simulink model "mini"  (R2023b)
settings: Solver=VariableStepAuto  StartTime=0.0  StopTime=10.0  RelTol=1e-3
libraries: arduinolib x9, arduinosensorlib x1
settings Model: Creator=yeoseojeong  LastModifiedBy=yeoseojeong

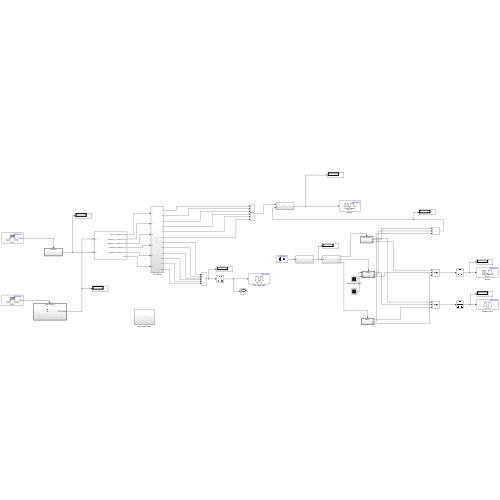
[thumbnail: Simulink's stored preview of the top-level diagram]
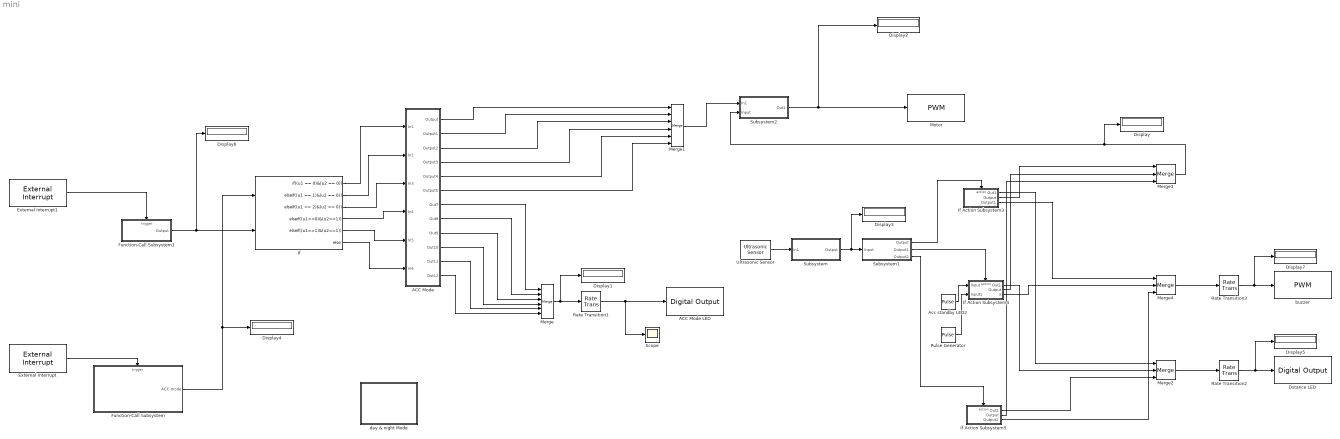
== system mini ==
  ACC Mode : Subsystem
  ACC Mode LED : arduinolib/Digital Output  pinNumber=12  Direction=output  blockPlatform=arduino
  Acc standby LED2 : DiscretePulseGenerator  PulseType=Time based  Period=0.4  PulseWidth=50
  Display{,1..7} (8 alike) : Display
  Dstance LED : arduinolib/Digital Output  pinNumber=13  Direction=output  blockPlatform=arduino
  External Interrupt : arduinolib/External Interrupt  Pin=2  PullUp=off  Mode=RISING  InterruptSimulationInput=off
  External Interrupt1 : arduinolib/External Interrupt  Pin=3  PullUp=off  Mode=RISING  InterruptSimulationInput=off
  Function-Call Subsystem : Subsystem  TreatAsAtomicUnit=on
  Function-Call Subsystem1 : Subsystem  TreatAsAtomicUnit=on
  If : If  NumInputs=2  IfExpression=(u1 == 0)&(u2 == 0)  ElseIfExpressions=(u1 == 1)&(u2 == 0),(u1 == 2)&(u2 == 0),(u1==0)&(u2==1),(u1==1)&(u2==1)
  If Action Subsystem3 : Subsystem  TreatAsAtomicUnit=on
  If Action Subsystem4 : Subsystem  TreatAsAtomicUnit=on
  If Action Subsystem5 : Subsystem  TreatAsAtomicUnit=on
  Merge : Merge  Inputs=6
  Merge1 : Merge  Inputs=6
  Merge2 : Merge  Inputs=3
  Merge3 : Merge  Inputs=3
  Merge4 : Merge  Inputs=3
  Motor : arduinolib/PWM  pinNumber=11  frequencyType=Default  desiredFrequency=490.2  achievableFrequency=490.2
  Pulse Generator : DiscretePulseGenerator  PulseType=Time based  Amplitude=200  PulseWidth=50
  Rate Transition1 : RateTransition  Deterministic=off
  Rate Transition2 : RateTransition  Deterministic=off
  Rate Transition3 : RateTransition  Deterministic=off
  Scope : Scope
  Subsystem : Subsystem
  Subsystem1 : Subsystem
  Subsystem2 : Subsystem
  Ultrasonic Sensor : arduinosensorlib/Ultrasonic Sensor  NumSignalPins=2  TrigPin=50  EchoPin=51  SignalPin=3  SampleTime_=1  blockPlatform=ARDUINO
  buzzer : arduinolib/PWM  pinNumber=5  frequencyType=Default  desiredFrequency=490.2  achievableFrequency=490.1961
  day & night Mode : Subsystem
  wires:
  ACC Mode/6(Output5) -> Merge1/6
  If Action Subsystem5/3(Output1) -> Merge4/3
  ACC Mode/7(Out7) -> Merge/1
  Merge4/1 -> Rate Transition3/1
  Rate Transition3/1 -> buzzer/1, Display7/1
  ACC Mode/8(Out8) -> Merge/2
  ACC Mode/10(Out10) -> Merge/4
  ACC Mode/1(Output) -> Merge1/1
  ACC Mode/12(Out12) -> Merge/6
  Merge2/1 -> Rate Transition2/1
  ACC Mode/9(Out9) -> Merge/3
  ACC Mode/5(Output4) -> Merge1/5
  If/3 -> ACC Mode/3(In3)
  Rate Transition1/1 -> ACC Mode LED/1, Scope/1
  ACC Mode/4(Output3) -> Merge1/4
  If/6 -> ACC Mode/6(In6)
  If/5 -> ACC Mode/5(In5)
  ACC Mode/2(Output1) -> Merge1/2
  If/4 -> ACC Mode/4(In4)
  Merge1/1 -> Subsystem2/1(In1)
  If Action Subsystem4/2(Output) -> Merge3/2
  External Interrupt/1 -> Function-Call Subsystem/Trigger
  If/2 -> ACC Mode/2(In2)
  If Action Subsystem4/3(Output1) -> Merge4/2
  If Action Subsystem3/3(Output1) -> Merge4/1
  Merge/1 -> Display1/1, Rate Transition1/1
  Function-Call Subsystem1/1(Output) -> Display6/1, If/2
  If Action Subsystem5/1(Out1) -> Merge2/3
  ACC Mode/3(Output2) -> Merge1/3
  Subsystem1/3(Output2) -> If Action Subsystem5/Action
  ACC Mode/11(Out11) -> Merge/5
  External Interrupt1/1 -> Function-Call Subsystem1/Trigger
  Pulse Generator/1 -> If Action Subsystem4/2(Input1)
  Acc standby LED2/1 -> If Action Subsystem4/1(Input)
  Merge3/1 -> Subsystem2/2(Input), Display/1
  Rate Transition2/1 -> Display5/1, Dstance LED/1
  If Action Subsystem3/2(Output) -> Merge3/1
  Subsystem1/2(Output1) -> If Action Subsystem4/Action
  Subsystem2/1(Out1) -> Display2/1, Motor/1
  If Action Subsystem3/1(Out1) -> Merge2/1
  Subsystem/1(Output) -> Subsystem1/1(Input), Display3/1
  If Action Subsystem4/1(Out1) -> Merge2/2
  Subsystem1/1(Output) -> If Action Subsystem3/Action
  If/1 -> ACC Mode/1(In1)
  Ultrasonic Sensor/1 -> Subsystem/1(In1)
  Function-Call Subsystem/1(ACC mode) -> Display4/1, If/1
  If Action Subsystem5/2(Output) -> Merge3/3

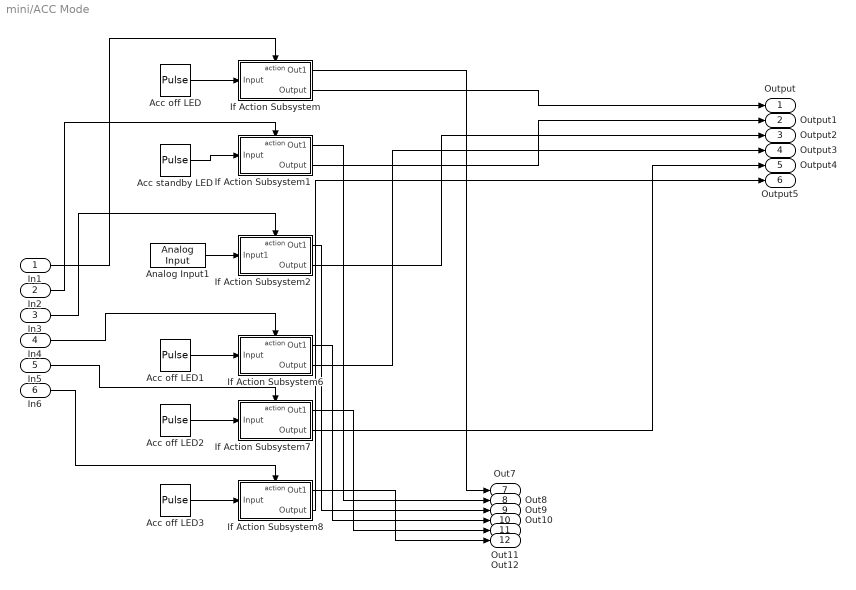
== system mini/ACC Mode ==
  In1 : Inport
  In2 : Inport  Port=2
  In3 : Inport  Port=3
  In4 : Inport  Port=4
  In5 : Inport  Port=5
  In6 : Inport  Port=6
  Acc off LED{,1..3} (4 alike) : DiscretePulseGenerator  PulseType=Time based  PulseWidth=50
  Acc standby LED : DiscretePulseGenerator  PulseType=Time based  Period=0.4  PulseWidth=50
  Analog Input1 : arduinolib/Analog Input  pinNumber=8  ReadResultsOnly=off  ConversionTriggerSource=Software  ExternalTriggerType=uint32( 0 )  OutputDataType=uint16  EnableConversionCompleteNotify=off  EnableOuputStatus=off  SampleTime=-1  blockPlatform=arduino
  If Action Subsystem : Subsystem  TreatAsAtomicUnit=on
  If Action Subsystem1 : Subsystem  TreatAsAtomicUnit=on
  If Action Subsystem2 : Subsystem  TreatAsAtomicUnit=on
  If Action Subsystem6 : Subsystem  TreatAsAtomicUnit=on
  If Action Subsystem7 : Subsystem  TreatAsAtomicUnit=on
  If Action Subsystem8 : Subsystem  TreatAsAtomicUnit=on
  Output : Outport
  Output1 : Outport  Port=2
  Output2 : Outport  Port=3
  Output3 : Outport  Port=4
  Output4 : Outport  Port=5
  Output5 : Outport  Port=6
  Out7 : Outport  Port=7
  Out8 : Outport  Port=8
  Out9 : Outport  Port=9
  Out10 : Outport  Port=10
  Out11 : Outport  Port=11
  Out12 : Outport  Port=12
  wires:
  In2/1 -> If Action Subsystem1/Action
  Acc off LED3/1 -> If Action Subsystem8/1(Input)
  Acc off LED/1 -> If Action Subsystem/1(Input)
  Acc standby LED/1 -> If Action Subsystem1/1(Input)
  If Action Subsystem1/2(Output) -> Output1/1
  If Action Subsystem8/1(Out1) -> Out12/1
  If Action Subsystem2/2(Output) -> Output2/1
  Acc off LED1/1 -> If Action Subsystem6/1(Input)
  Acc off LED2/1 -> If Action Subsystem7/1(Input)
  If Action Subsystem8/2(Output) -> Output5/1
  In3/1 -> If Action Subsystem2/Action
  Analog Input1/1 -> If Action Subsystem2/1(Input1)
  In1/1 -> If Action Subsystem/Action
  If Action Subsystem/1(Out1) -> Out7/1
  If Action Subsystem1/1(Out1) -> Out8/1
  In4/1 -> If Action Subsystem6/Action
  If Action Subsystem6/2(Output) -> Output3/1
  In6/1 -> If Action Subsystem8/Action
  If Action Subsystem/2(Output) -> Output/1
  If Action Subsystem6/1(Out1) -> Out10/1
  If Action Subsystem7/2(Output) -> Output4/1
  If Action Subsystem7/1(Out1) -> Out11/1
  In5/1 -> If Action Subsystem7/Action
  If Action Subsystem2/1(Out1) -> Out9/1

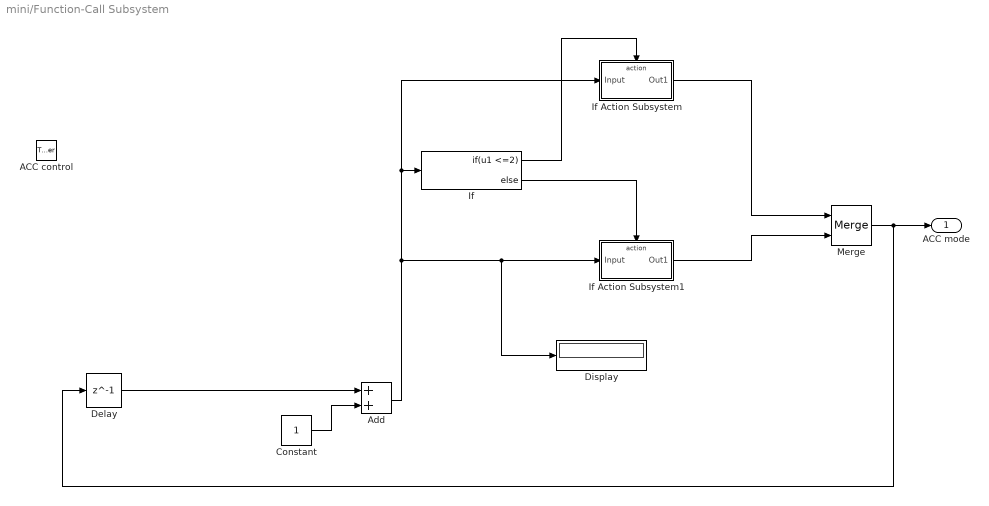
== system mini/Function-Call Subsystem ==
  ACC control : TriggerPort  TriggerType=function-call  VariantControl=(inherit)
  Add : Sum
  Constant : Constant
  Delay : Delay  DelayLength=1
  Display : Display
  If : If  IfExpression=u1 <=2
  If Action Subsystem : Subsystem  TreatAsAtomicUnit=on
  If Action Subsystem1 : Subsystem  TreatAsAtomicUnit=on
  Merge : Merge
  ACC mode : Outport
  wires:
  Delay/1 -> Add/1
  Constant/1 -> Add/2
  If/1 -> If Action Subsystem/Action
  If/2 -> If Action Subsystem1/Action
  If Action Subsystem/1(Out1) -> Merge/1
  If Action Subsystem1/1(Out1) -> Merge/2
  Add/1 -> If Action Subsystem/1(Input), If/1, Display/1, If Action Subsystem1/1(Input)
  Merge/1 -> Delay/1, ACC mode/1

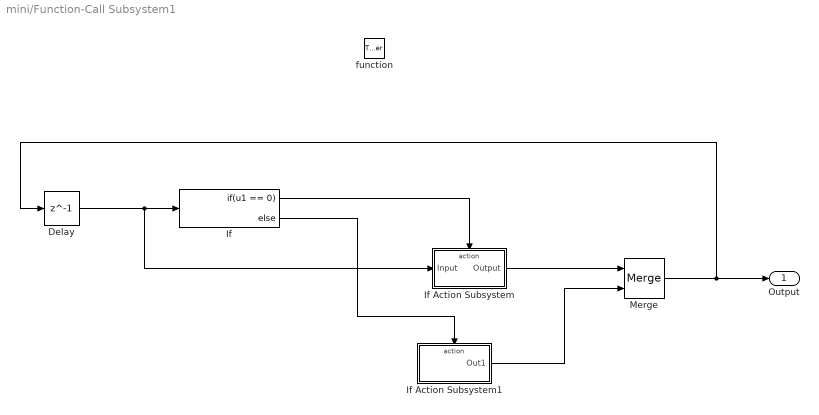
== system mini/Function-Call Subsystem1 ==
  function : TriggerPort  TriggerType=function-call  VariantControl=(inherit)
  Delay : Delay  DelayLength=1
  If : If  IfExpression=u1 == 0
  If Action Subsystem : Subsystem  TreatAsAtomicUnit=on
  If Action Subsystem1 : Subsystem  TreatAsAtomicUnit=on
  Merge : Merge
  Output : Outport
  wires:
  Delay/1 -> If Action Subsystem/1(Input), If/1
  If/1 -> If Action Subsystem/Action
  If Action Subsystem/1(Output) -> Merge/1
  If/2 -> If Action Subsystem1/Action
  If Action Subsystem1/1(Out1) -> Merge/2
  Merge/1 -> Delay/1, Output/1

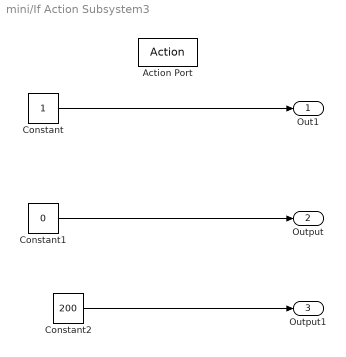
== system mini/If Action Subsystem3 ==
  Action Port : ActionPort  ActionPortLabel=if(u1 <= 200)
  Constant : Constant
  Constant1 : Constant  Value=0
  Constant2 : Constant  Value=200
  Out1 : Outport
  Output : Outport  Port=2
  Output1 : Outport  Port=3
  wires:
  Constant/1 -> Out1/1
  Constant1/1 -> Output/1
  Constant2/1 -> Output1/1

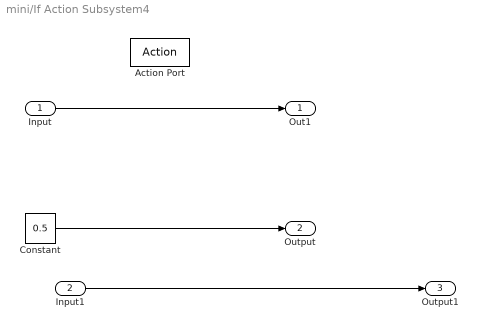
== system mini/If Action Subsystem4 ==
  Input : Inport
  Input1 : Inport  Port=2
  Action Port : ActionPort  ActionPortLabel=elseif(..)
  Constant : Constant  Value=0.5
  Out1 : Outport
  Output : Outport  Port=2
  Output1 : Outport  Port=3
  wires:
  Input/1 -> Out1/1
  Constant/1 -> Output/1
  Input1/1 -> Output1/1

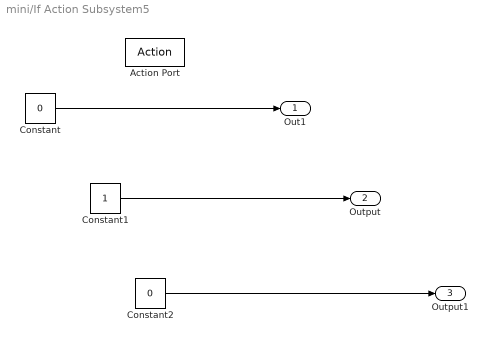
== system mini/If Action Subsystem5 ==
  Action Port : ActionPort  ActionPortLabel=else
  Constant : Constant  Value=0
  Constant1 : Constant
  Constant2 : Constant  Value=0
  Out1 : Outport
  Output : Outport  Port=2
  Output1 : Outport  Port=3
  wires:
  Constant/1 -> Out1/1
  Constant1/1 -> Output/1
  Constant2/1 -> Output1/1

== system mini/Subsystem ==
  In1 : Inport
  Constant : Constant  Value=2
  Constant1 : Constant  Value=3400
  Divide : Product  Inputs=**
  Divide1 : Product  Inputs=*/
  Output : Outport
  wires:
  Constant1/1 -> Divide/2
  Divide/1 -> Divide1/1
  Constant/1 -> Divide1/2
  Divide1/1 -> Output/1
  In1/1 -> Divide/1

== system mini/Subsystem1 ==
  Input : Inport
  If : If  IfExpression=u1 <= 200  ElseIfExpressions=(u1>=250)&(u1<=800)
  Output : Outport
  Output1 : Outport  Port=2
  Output2 : Outport  Port=3
  wires:
  Input/1 -> If/1
  If/1 -> Output/1
  If/2 -> Output1/1
  If/3 -> Output2/1

== system mini/Subsystem2 ==
  In1 : Inport
  Input : Inport  Port=2
  Divide : Product  Inputs=**
  Out1 : Outport
  wires:
  In1/1 -> Divide/1
  Input/1 -> Divide/2
  Divide/1 -> Out1/1

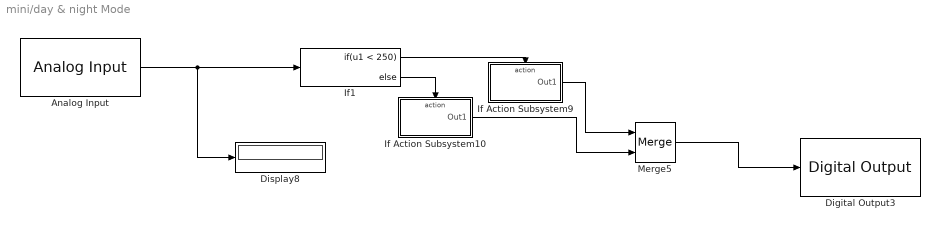
== system mini/day & night Mode ==
  Analog Input : arduinolib/Analog Input  pinNumber=10  ReadResultsOnly=off  ConversionTriggerSource=Software  ExternalTriggerType=uint32( 0 )  OutputDataType=uint16  EnableConversionCompleteNotify=off  EnableOuputStatus=off  SampleTime=-1  blockPlatform=arduino
  Digital Output3 : arduinolib/Digital Output  pinNumber=30  Direction=output  blockPlatform=arduino
  Display8 : Display
  If Action Subsystem10 : Subsystem  TreatAsAtomicUnit=on
  If Action Subsystem9 : Subsystem  TreatAsAtomicUnit=on
  If1 : If  IfExpression=u1 < 250
  Merge5 : Merge
  wires:
  If Action Subsystem10/1(Out1) -> Merge5/2
  If1/2 -> If Action Subsystem10/Action
  Analog Input/1 -> Display8/1, If1/1
  If Action Subsystem9/1(Out1) -> Merge5/1
  If1/1 -> If Action Subsystem9/Action
  Merge5/1 -> Digital Output3/1

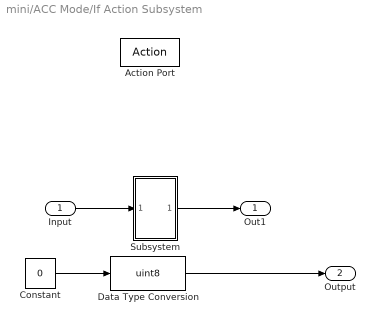
== system mini/ACC Mode/If Action Subsystem ==
  Input : Inport
  Action Port : ActionPort  ActionPortLabel=if((u1 == 0)&(u2 == 0))
  Constant : Constant  Value=0
  Data Type Conversion : DataTypeConversion  OutDataTypeStr=uint8  SaturateOnIntegerOverflow=off  RndMeth=Floor
  Subsystem : Subsystem
  Out1 : Outport
  Output : Outport  Port=2
  wires:
  Constant/1 -> Data Type Conversion/1
  Data Type Conversion/1 -> Output/1
  Input/1 -> Subsystem/1(Input)
  Subsystem/1(Out1) -> Out1/1

== system mini/ACC Mode/If Action Subsystem1 ==
  Input : Inport
  Action Port : ActionPort  ActionPortLabel=elseif((u1 == 1)&(u2 == 0))
  Constant : Constant  Value=120
  Data Type Conversion : DataTypeConversion  OutDataTypeStr=uint8  SaturateOnIntegerOverflow=off  RndMeth=Floor
  Out1 : Outport
  Output : Outport  Port=2
  wires:
  Input/1 -> Out1/1
  Data Type Conversion/1 -> Output/1
  Constant/1 -> Data Type Conversion/1

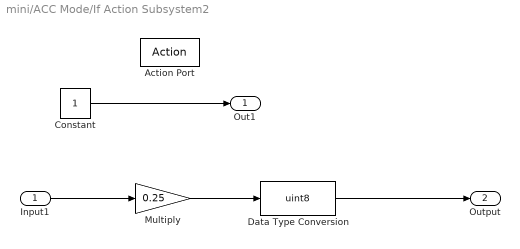
== system mini/ACC Mode/If Action Subsystem2 ==
  Input1 : Inport
  Action Port : ActionPort  ActionPortLabel=elseif((u1 == 2)&(u2 == 0))
  Constant : Constant
  Data Type Conversion : DataTypeConversion  OutDataTypeStr=uint8  SaturateOnIntegerOverflow=off  RndMeth=Floor
  Multiply : Gain  Gain=0.25
  Out1 : Outport
  Output : Outport  Port=2
  wires:
  Constant/1 -> Out1/1
  Input1/1 -> Multiply/1
  Multiply/1 -> Data Type Conversion/1
  Data Type Conversion/1 -> Output/1

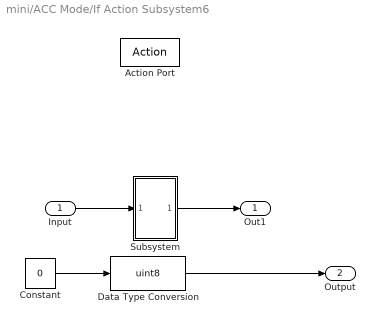
== system mini/ACC Mode/If Action Subsystem6 ==
  Input : Inport
  Action Port : ActionPort  ActionPortLabel=elseif((u1==0)&(u2==1))
  Constant : Constant  Value=0
  Data Type Conversion : DataTypeConversion  OutDataTypeStr=uint8  SaturateOnIntegerOverflow=off  RndMeth=Floor
  Subsystem : Subsystem
  Out1 : Outport
  Output : Outport  Port=2
  wires:
  Constant/1 -> Data Type Conversion/1
  Data Type Conversion/1 -> Output/1
  Input/1 -> Subsystem/1(Input)
  Subsystem/1(Out1) -> Out1/1

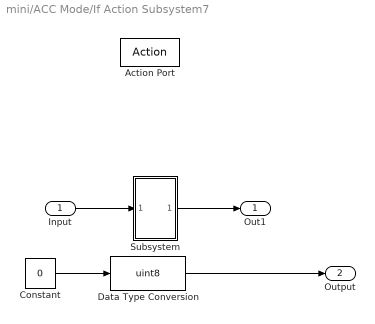
== system mini/ACC Mode/If Action Subsystem7 ==
  Input : Inport
  Action Port : ActionPort  ActionPortLabel=elseif((u1==1)&(u2==1))
  Constant : Constant  Value=0
  Data Type Conversion : DataTypeConversion  OutDataTypeStr=uint8  SaturateOnIntegerOverflow=off  RndMeth=Floor
  Subsystem : Subsystem
  Out1 : Outport
  Output : Outport  Port=2
  wires:
  Constant/1 -> Data Type Conversion/1
  Data Type Conversion/1 -> Output/1
  Input/1 -> Subsystem/1(Input)
  Subsystem/1(Out1) -> Out1/1

== system mini/ACC Mode/If Action Subsystem8 ==
  Input : Inport
  Action Port : ActionPort  ActionPortLabel=else
  Constant : Constant  Value=0
  Data Type Conversion : DataTypeConversion  OutDataTypeStr=uint8  SaturateOnIntegerOverflow=off  RndMeth=Floor
  Subsystem : Subsystem
  Out1 : Outport
  Output : Outport  Port=2
  wires:
  Constant/1 -> Data Type Conversion/1
  Data Type Conversion/1 -> Output/1
  Input/1 -> Subsystem/1(Input)
  Subsystem/1(Out1) -> Out1/1

== system mini/Function-Call Subsystem/If Action Subsystem ==
  Input : Inport
  Action Port : ActionPort  ActionPortLabel=if(u1 <=2)
  Out1 : Outport
  wires:
  Input/1 -> Out1/1

== system mini/Function-Call Subsystem/If Action Subsystem1 ==
  Input : Inport
  Action Port : ActionPort  ActionPortLabel=else
  Constant : Constant  Value=0
  Divide : Product  Inputs=**
  Out1 : Outport
  wires:
  Divide/1 -> Out1/1
  Constant/1 -> Divide/1
  Input/1 -> Divide/2

== system mini/Function-Call Subsystem1/If Action Subsystem ==
  Input : Inport
  Action Port : ActionPort  ActionPortLabel=if(u1 == 0)
  Add : Sum
  Constant : Constant
  Output : Outport
  wires:
  Add/1 -> Output/1
  Input/1 -> Add/1
  Constant/1 -> Add/2

== system mini/Function-Call Subsystem1/If Action Subsystem1 ==
  Action Port : ActionPort  ActionPortLabel=else
  Constant : Constant  Value=0
  Out1 : Outport
  wires:
  Constant/1 -> Out1/1

== system mini/day & night Mode/If Action Subsystem10 ==
  Action Port : ActionPort  ActionPortLabel=else
  Constant : Constant  Value=0
  Out1 : Outport
  wires:
  Constant/1 -> Out1/1

== system mini/day & night Mode/If Action Subsystem9 ==
  Action Port : ActionPort  ActionPortLabel=if(u1 < 250)
  Constant : Constant
  Out1 : Outport
  wires:
  Constant/1 -> Out1/1

== system mini/ACC Mode/If Action Subsystem/Subsystem ==
  Input : Inport
  Out1 : Outport
  wires:
  Input/1 -> Out1/1

== system mini/ACC Mode/If Action Subsystem6/Subsystem ==
  Input : Inport
  Out1 : Outport
  wires:
  Input/1 -> Out1/1

== system mini/ACC Mode/If Action Subsystem7/Subsystem ==
  Input : Inport
  Out1 : Outport
  wires:
  Input/1 -> Out1/1

== system mini/ACC Mode/If Action Subsystem8/Subsystem ==
  Input : Inport
  Out1 : Outport
  wires:
  Input/1 -> Out1/1
